simulink model "Part_B"  (R2021b)
settings: Solver=VariableStepAuto  StartTime=0.0  StopTime=2/1000  RelTol=1e-3
values from neighbouring files (symbols this model uses):
  kf = 6000    [Gen_Workspace_vars.m]    (also in Part_A.m = 2000)
undefined symbols (not defined in the file or in its folder): DiscIntNeverNeededParam
settings Model: Creator=Youssef Islam  LastModifiedBy=Youssef Islam

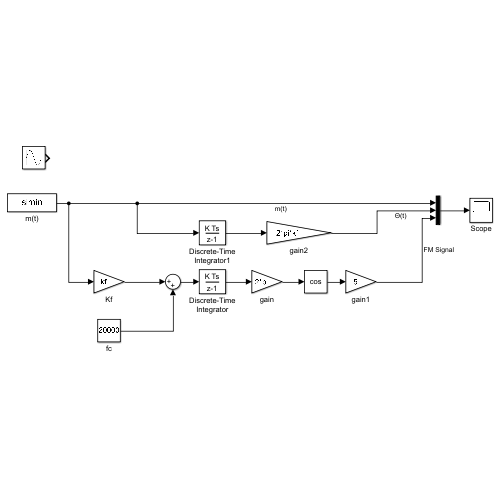
[thumbnail: Simulink's stored preview of the top-level diagram]
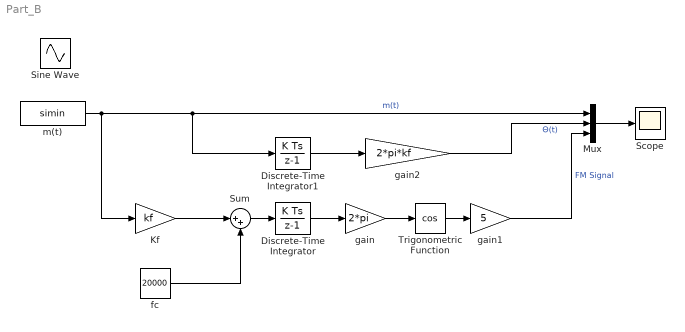
== system Part_B ==
  Discrete-Time Integrator : DiscreteIntegrator  SampleTime=0.0000001  ICPrevOutput=DiscIntNeverNeededParam  ICPrevScaledInput=DiscIntNeverNeededParam
  Discrete-Time Integrator1 : DiscreteIntegrator  SampleTime=0.0000001  ICPrevOutput=DiscIntNeverNeededParam  ICPrevScaledInput=DiscIntNeverNeededParam
  Kf : Gain  Description=Kp=2000  Gain=kf
  Mux : Mux  Inputs=3
  Scope : Scope
  Sine Wave : Sin  Amplitude=3  Frequency=2*pi*1000  SampleTime=0
  Sum : Sum  Inputs=|++
  Trigonometric Function : Trigonometry  Operator=cos
  fc : Constant  Value=20000
  gain : Gain  Description=Kp=2000  Gain=2*pi
  gain1 : Gain  Description=Kp=2000  Gain=5
  gain2 : Gain  Description=Kp=2000  Gain=2*pi*kf
  m(t) : FromWorkspace  VariableName=simin
  wires:
  Mux/1 -> Scope/1
  m(t)/1 -> Kf/1, Discrete-Time Integrator1/1, Mux/1  "m(t)"
  Kf/1 -> Sum/1
  fc/1 -> Sum/2
  gain/1 -> Trigonometric Function/1
  Trigonometric Function/1 -> gain1/1
  gain1/1 -> Mux/3  "FM Signal"
  Sum/1 -> Discrete-Time Integrator/1
  Discrete-Time Integrator/1 -> gain/1
  Discrete-Time Integrator1/1 -> gain2/1
  gain2/1 -> Mux/2  "Θ(t)"
